simulink model "Q2_b2"  (R2015a)
settings: Solver=ode45  StartTime=0.0  StopTime=2  RelTol=1e-10  AbsTol=1e-10
libraries: cstblocks x4
settings Model: Creator=yarde_000  LastModifiedBy=yarde_000

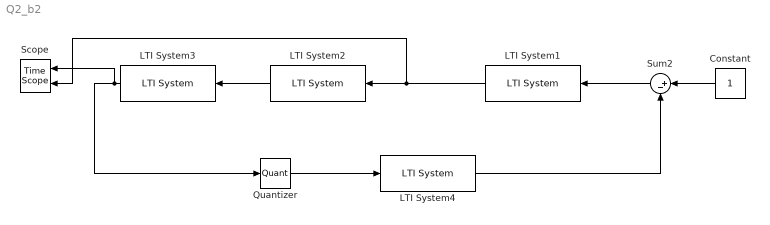
== system Q2_b2 ==
  Constant : Constant
  LTI System1 : cstblocks/LTI System  sys=C  IC=[]
  LTI System2 : cstblocks/LTI System  sys=P  IC=[]
  LTI System3 : cstblocks/LTI System  sys=tf(1, [1 0])  IC=[]
  LTI System4 : cstblocks/LTI System  sys=H  IC=[]
  Quantizer : Quantizer  QuantizationInterval=enc_res
  Scope : TimeScope  NumInputPorts=2
  Sum2 : Sum  Inputs=|+-
  wires:
  Sum2/1 -> LTI System1/1
  LTI System2/1 -> LTI System3/1
  LTI System3/1 -> Quantizer/1, Scope/1
  Constant/1 -> Sum2/1
  Quantizer/1 -> LTI System4/1
  LTI System4/1 -> Sum2/2
  LTI System1/1 -> Scope/2, LTI System2/1
